simulink model "ax_plus_b"  (R2024a)
settings: Solver=VariableStepAuto  StartTime=0.0  StopTime=10.0  RelTol=1e-3
values from neighbouring files (symbols this model uses):
  a = 10    [test_script.m]
  b = 20    [test_script.m]
settings Model: Creator=Lenovo  LastModifiedBy=Lenovo

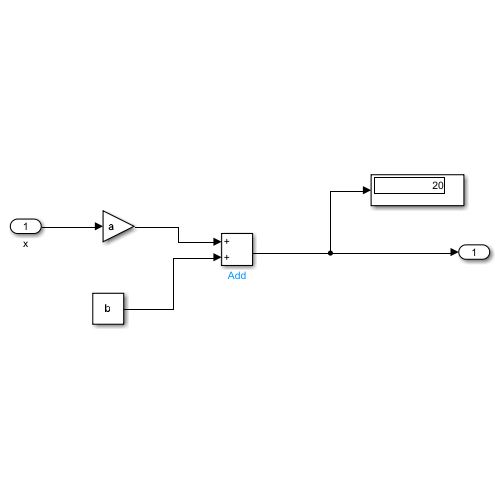
[thumbnail: Simulink's stored preview of the top-level diagram]
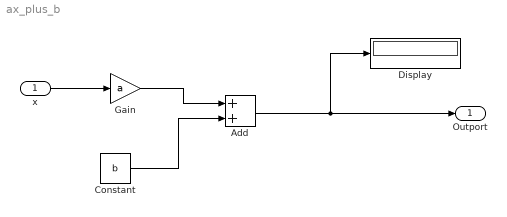
== system ax_plus_b ==
  x : Inport
  Add : Sum
  Constant : Constant  Value=b
  Display : Display
  Gain : Gain  Gain=a
  Outport : Outport
  wires:
  x/1 -> Gain/1
  Add/1 -> Display/1, Outport/1
  Gain/1 -> Add/1
  Constant/1 -> Add/2
